simulink model "ndtm_V2"  (R2018b)
settings: configuration reference "Physics" (kept outside this file)
model workspace (MAT data in the model file):
  x0_initialstates = [0 0 0 0 0 0]
undefined symbols (not defined in the file): F0z, h, INIT__initialvalues__Vehicle_InitialPitchRate_radps, INIT__initialvalues__Vehicle_InitialRollRate_radps, INIT__initialvalues__Vehicle_InitialVelocity_mps__1, INIT__initialvalues__Vehicle_InitialVelocity_mps__2, INIT__initialvalues__Vehicle_InitialVelocity_mps__3, INIT__initialvalues__Vehicle_InitialYawRate_radps, SUS__Antisway__c_AntiSwayTSpringFrRe_Nmprad__1, SUS__Antisway__c_AntiSwayTSpringFrRe_Nmprad__2, SUS__Antisway__phi_AntiSwayNeutralAngleFrRe_rad__1, SUS__Antisway__phi_AntiSwayNeutralAngleFrRe_rad__2, SUS__Antisway__r_AntiSwayArmRadiusFrRe_m__1, SUS__Antisway__r_AntiSwayArmRadiusFrRe_m__2, SUS__Compliance__Cz_DamperRateFrRe_Nspm__1, SUS__Compliance__Cz_DamperRateFrRe_Nspm__2, SUS__Compliance__cz_SpringRateFrRe_Npm__1, SUS__Compliance__cz_SpringRateFrRe_Npm__2, SUS__Compliance__F0z_SpringPreloadFrRe_N__1, SUS__Compliance__F0z_SpringPreloadFrRe_N__2, SUS__Compliance__h_InertialFrameOffset_COGtoAxle_m, SUS__Kinematics__k_CamberATSteerCenterF__1, SUS__Kinematics__k_CamberATSteerCenterF__2, SUS__Kinematics__k_CamberVSHeightFrRe__1, SUS__Kinematics__k_CamberVSHeightFrRe__2, SUS__Kinematics__k_CasterATSteerCenterF__1, SUS__Kinematics__k_CasterATSteerCenterF__2, SUS__Kinematics__k_CasterVSHeightFrRe__1, SUS__Kinematics__k_CasterVSHeightFrRe__2, SUS__Kinematics__k_RollSteerVSHeightFrRe_radpm__1, SUS__Kinematics__k_RollSteerVSHeightFrRe_radpm__2, SUS__Kinematics__nu0_ToeATSteerCenterFrRe_rad__1, SUS__Kinematics__nu0_ToeATSteerCenterFrRe_rad__2, tireFL__SCALING__LFZO, tireFR__SCALING__LFZO, tireRL__SCALING__LFZO, tireRR__SCALING__LFZO, VEH, VEH__Aerodynamics__beta_wind_end_rad, VEH__Aerodynamics__beta_wind_start_rad, VEH__Aerodynamics__beta_wind_step_rad, VEH__Aerodynamics__cl_LongitudinalLift, VEH__Aerodynamics__Cs_LatDragCoeff_end, VEH__Aerodynamics__Cs_LatDragCoeff_start, VEH__Aerodynamics__Cs_LatDragCoeff_step, VEH__Aerodynamics__Cym_DragYawMomentCoeff_end, VEH__Aerodynamics__Cym_DragYawMomentCoeff_start, VEH__Aerodynamics__Cym_DragYawMomentCoeff_step, VEH__Environment__a_Gravity_mps2, VEH__Tires__p_Tires_pa__1, VEH__Tires__p_Tires_pa__2, VEH__Tires__p_Tires_pa__3, VEH__Tires__p_Tires_pa__4, VEH__VehicleData__l_WheelbaseF_m, VEH__VehicleData__l_WheelbaseTotal_m, VEH__VehicleData__m_Vehicle_kg, VEH__VehicleData__w_GeomCenterlineToCOG_m, VEH__VehicleData__w_TrackF_m, VEH__VehicleData__w_TrackR_m
libraries: vehdynlibsuspension x7, vehdynlibtire x4, vehdynlibtire_TUM x4, autolibutils x2, sharedtransform x2, vehdynlibeom_TUM x1
(part 1 of 4)
settings Model: DataDictionary=vehicleparameters_vehdynsim.sldd  ModifiedByFormat=The MathWorks, Inc.  ParameterArgumentNames=x0_initialstates  OrderedModelArguments=off  Creator=The MathWorks, Inc.  LastModifiedBy=The MathWorks, Inc.

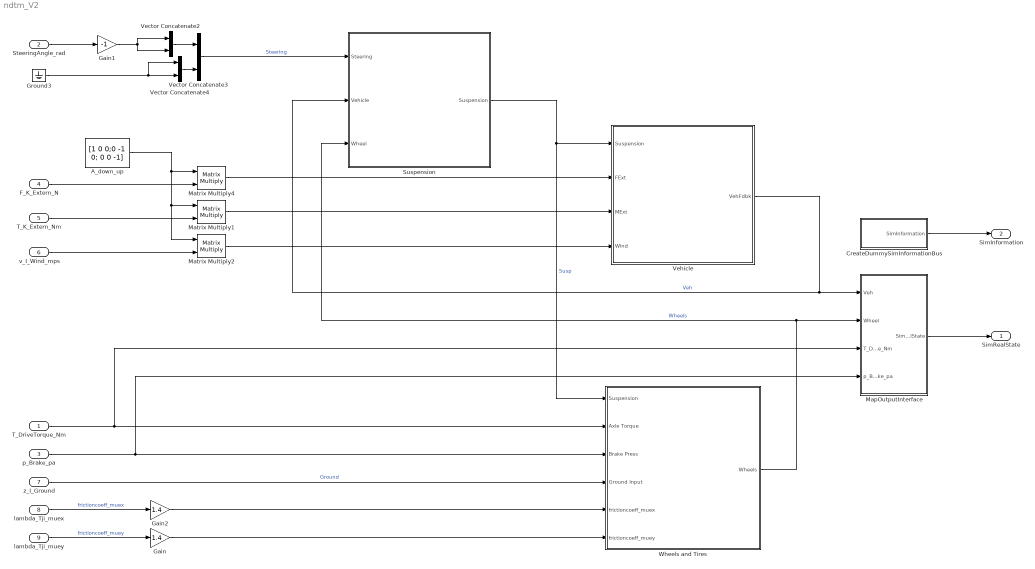
== system ndtm_V2 ==
  T_DriveTorque_Nm : Inport
  SteeringAngle_rad : Inport  Port=2
  p_Brake_pa : Inport  Port=3
  F_K_Extern_N : Inport  Port=4  PortDimensions=3
  T_K_Extern_Nm : Inport  Port=5  PortDimensions=3
  v_I_Wind_mps : Inport  Port=6  PortDimensions=3
  z_I_Ground : Inport  Port=7  PortDimensions=4
  lambda_Tji_muex : Inport  Port=8  PortDimensions=4
  lambda_Tji_muey : Inport  Port=9  PortDimensions=4
  A_down_up : Constant  Value=[1 0 0;0 -1 0; 0 0 -1]
  CreateDummySimInformationBus : Subsystem
  Gain : Gain  Gain=1.4
  Gain1 : Gain  Gain=-1
  Gain2 : Gain  Gain=1.4
  Ground3 : Ground
  MapOutputInterface : Subsystem
  Matrix Multiply1 : Product  Multiplication=Matrix(*)
  Matrix Multiply2 : Product  Multiplication=Matrix(*)
  Matrix Multiply4 : Product  Multiplication=Matrix(*)
  Suspension : Subsystem  VariantControlMode=Label  Variant=on  LabelModeActiveChoice=1
      mask Display:
      | switch str2num(get_param(gcb,'ActiveVariant'))
      |     case 1
      |         image('suspdw.png');
      |     case 2
      |         image([imread('suspindmap.png');imread('suspsamap.png')]);
      |     case 3
      |          image([imread('suspmacp.png');imread('suspsacoil.png')]);
      |     case 4
      |          image('suspmacp.png');
      |     case 5
      |          image('suspindmap.png');
      | end
  Vector Concatenate2 : Concatenate
  Vector Concatenate3 : Concatenate
  Vector Concatenate4 : Concatenate
  Vehicle : Subsystem
      mask Display: image('6dofcar.png');
  Wheels and Tires : Subsystem
      mask Display: image('wheel3dof.png')
  SimRealState : Outport  OutDataTypeStr=Bus: SimRealState
  SimInformation : Outport  Port=2  OutDataTypeStr=Bus: SimInformation
  wires:
  Vehicle/1(VehFdbk) -> Suspension/2(Vehicle), MapOutputInterface/1(Veh)  "Veh"
  Vector Concatenate3/1 -> Suspension/1(Steering)  "Steering"
  Suspension/1(Suspension) -> Vehicle/1(Suspension), Wheels and Tires/1(Suspension)  "Susp"
  Wheels and Tires/1(Wheels) -> MapOutputInterface/2(Wheel), Suspension/3(Wheel)  "Wheels"
  z_I_Ground/1 -> Wheels and Tires/4(Ground Input)  "Ground"
  p_Brake_pa/1 -> Wheels and Tires/3(Brake Press), MapOutputInterface/4("p_Brake_pa ")
  Ground3/1 -> Vector Concatenate4/1, Vector Concatenate4/2
  lambda_Tji_muey/1 -> Gain/1  "frictioncoeff_muey"
  Gain1/1 -> Vector Concatenate2/2, Vector Concatenate2/1
  Matrix Multiply4/1 -> Vehicle/2(FExt)
  Vector Concatenate2/1 -> Vector Concatenate3/1
  Matrix Multiply2/1 -> Vehicle/4(Wind)
  Matrix Multiply1/1 -> Vehicle/3(MExt)
  Vector Concatenate4/1 -> Vector Concatenate3/2
  T_DriveTorque_Nm/1 -> Wheels and Tires/2(Axle Torque), MapOutputInterface/3(T_DriveTorque_Nm)
  CreateDummySimInformationBus/1(SimInformation) -> SimInformation/1
  MapOutputInterface/1(SimRealState) -> SimRealState/1
  SteeringAngle_rad/1 -> Gain1/1
  lambda_Tji_muex/1 -> Gain2/1  "frictioncoeff_muex"
  F_K_Extern_N/1 -> Matrix Multiply4/2
  A_down_up/1 -> Matrix Multiply2/1, Matrix Multiply1/1, Matrix Multiply4/1
  T_K_Extern_Nm/1 -> Matrix Multiply1/2
  v_I_Wind_mps/1 -> Matrix Multiply2/2
  Gain2/1 -> Wheels and Tires/5(frictioncoeff_muex)
  Gain/1 -> Wheels and Tires/6(frictioncoeff_muey)

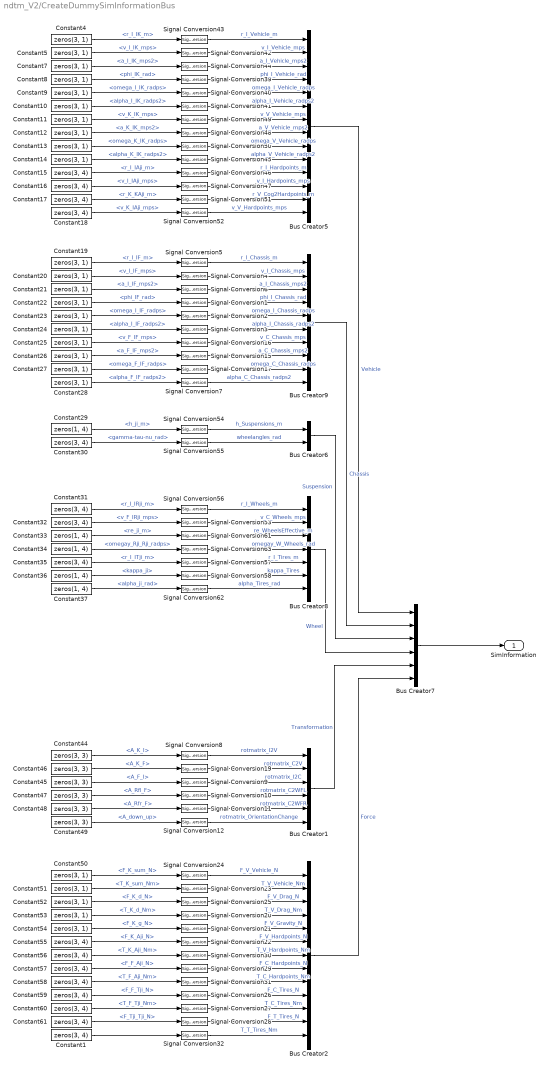
== system ndtm_V2/CreateDummySimInformationBus ==
  Bus Creator1 : BusCreator  Inputs=6  OutDataTypeStr=Bus: Transformation
      settings: InheritFromInputs=off
  Bus Creator2 : BusCreator  Inputs=13  OutDataTypeStr=Bus: Force
      settings: InheritFromInputs=off
  Bus Creator5 : BusCreator  Inputs=14  OutDataTypeStr=Bus: Vehicle
      settings: InheritFromInputs=off
  Bus Creator6 : BusCreator  Inputs=2  OutDataTypeStr=Bus: Suspension
      settings: InheritFromInputs=off
  Bus Creator7 : BusCreator  Inputs=6  OutDataTypeStr=Bus: SimInformation
      settings: InheritFromInputs=off
  Bus Creator8 : BusCreator  Inputs=7  OutDataTypeStr=Bus: Wheel
      settings: InheritFromInputs=off
  Bus Creator9 : BusCreator  Inputs=10  OutDataTypeStr=Bus: Chassis
      settings: InheritFromInputs=off
  Constant{1,15..18,30..32,35,55..61} (16 alike) : Constant  Value=zeros(3, 4)
  Constant{4..5,7..14,19..28,50..54} (25 alike) : Constant  Value=zeros(3, 1)
  Constant{29,33..34,36..37} (5 alike) : Constant  Value=zeros(1, 4)
  Constant{44..49} (6 alike) : Constant  Value=zeros(3, 3)
  Signal Conversion{1..12,15..17,19..32,39..58,61..63} (52 alike) : SignalConversion  OverrideOpt=off
  SimInformation : Outport  OutDataTypeStr=Bus: SimInformation
  wires:
  Signal Conversion46/1 -> Bus Creator5/11  "r_I_Hardpoints_m"
  Signal Conversion26/1 -> Bus Creator2/10  "F_C_Tires_N"
  Signal Conversion45/1 -> Bus Creator5/10  "alpha_V_Vehicle_radps2"
  Constant33/1 -> Signal Conversion61/1  "<re_ji_m>"
  Signal Conversion15/1 -> Bus Creator9/8  "a_C_Chassis_mps2"
  Signal Conversion58/1 -> Bus Creator8/6  "kappa_Tires"
  Constant60/1 -> Signal Conversion27/1  "<T_F_Tji_Nm>"
  Signal Conversion5/1 -> Bus Creator9/1  "r_I_Chassis_m"
  Signal Conversion17/1 -> Bus Creator9/9  "omega_C_Chassis_radps"
  Signal Conversion8/1 -> Bus Creator1/1  "rotmatrix_I2V"
  Constant13/1 -> Signal Conversion50/1  "<omega_K_IK_radps>"
  Constant24/1 -> Signal Conversion3/1  "<alpha_I_IF_radps2>"
  Signal Conversion16/1 -> Bus Creator9/7  "v_C_Chassis_mps"
  Signal Conversion23/1 -> Bus Creator2/2  "T_V_Vehicle_Nm"
  Signal Conversion3/1 -> Bus Creator9/6  "alpha_I_Chassis_radps2"
  Bus Creator5/1 -> Bus Creator7/1  "Vehicle"
  Signal Conversion32/1 -> Bus Creator2/13  "T_T_Tires_Nm"
  Signal Conversion39/1 -> Bus Creator5/4  "phi_I_Vehicle_rad"
  Signal Conversion29/1 -> Bus Creator2/8  "F_C_Hardpoints_N"
  Constant25/1 -> Signal Conversion16/1  "<v_F_IF_mps>"
  Signal Conversion43/1 -> Bus Creator5/1  "r_I_Vehicle_m"
  Constant47/1 -> Signal Conversion10/1  "<A_Rfl_F>"
  Constant9/1 -> Signal Conversion40/1  "<omega_I_IK_radps>"
  Constant26/1 -> Signal Conversion15/1  "<a_F_IF_mps2>"
  Constant27/1 -> Signal Conversion17/1  "<omega_F_IF_radps>"
  Signal Conversion10/1 -> Bus Creator1/4  "rotmatrix_C2WFL"
  Signal Conversion19/1 -> Bus Creator1/2  "rotmatrix_C2V"
  Constant7/1 -> Signal Conversion44/1  "<a_I_IK_mps2>"
  Bus Creator8/1 -> Bus Creator7/4  "Wheel"
  Signal Conversion9/1 -> Bus Creator1/3  "rotmatrix_I2C"
  Signal Conversion31/1 -> Bus Creator2/9  "T_C_Hardpoints_Nm"
  Signal Conversion62/1 -> Bus Creator8/7  "alpha_Tires_rad"
  Signal Conversion30/1 -> Bus Creator2/7  "T_V_Hardpoints_Nm"
  Signal Conversion48/1 -> Bus Creator5/8  "a_V_Vehicle_mps2"
  Signal Conversion54/1 -> Bus Creator6/1  "h_Suspensions_m"
  Signal Conversion56/1 -> Bus Creator8/1  "r_I_Wheels_m"
  Signal Conversion7/1 -> Bus Creator9/10  "alpha_C_Chassis_radps2"
  Signal Conversion12/1 -> Bus Creator1/6  "rotmatrix_OrientationChange"
  Signal Conversion21/1 -> Bus Creator2/5  "F_V_Gravity_N"
  Signal Conversion53/1 -> Bus Creator8/2  "v_C_Wheels_mps"
  Signal Conversion22/1 -> Bus Creator2/6  "F_V_Hardpoints_N"
  Signal Conversion27/1 -> Bus Creator2/11  "T_C_Tires_Nm"
  Signal Conversion51/1 -> Bus Creator5/13  "r_V_Cog2Hardpoints_m"
  Constant28/1 -> Signal Conversion7/1  "<alpha_F_IF_radps2>"
  Signal Conversion55/1 -> Bus Creator6/2  "wheelangles_rad"
  Signal Conversion57/1 -> Bus Creator8/5  "r_I_Tires_m"
  Signal Conversion4/1 -> Bus Creator9/2  "v_I_Chassis_mps"
  Bus Creator2/1 -> Bus Creator7/6  "Force"
  Signal Conversion20/1 -> Bus Creator2/4  "T_V_Drag_Nm"
  Signal Conversion40/1 -> Bus Creator5/5  "omega_I_Vehicle_radps"
  Bus Creator1/1 -> Bus Creator7/5  "Transformation"
  Signal Conversion41/1 -> Bus Creator5/6  "alpha_I_Vehicle_radps2"
  Bus Creator9/1 -> Bus Creator7/2  "Chassis"
  Signal Conversion6/1 -> Bus Creator9/3  "a_I_Chassis_mps2"
  Bus Creator6/1 -> Bus Creator7/3  "Suspension"
  Signal Conversion61/1 -> Bus Creator8/3  "re_WheelsEffective_m"
  Signal Conversion44/1 -> Bus Creator5/3  "a_I_Vehicle_mps2"
  Signal Conversion42/1 -> Bus Creator5/2  "v_I_Vehicle_mps"
  Signal Conversion63/1 -> Bus Creator8/4  "omegay_W_Wheels_rad"
  Constant31/1 -> Signal Conversion56/1  "<r_I_IRji_m>"
  Signal Conversion49/1 -> Bus Creator5/7  "v_V_Vehicle_mps"
  Signal Conversion28/1 -> Bus Creator2/12  "F_T_Tires_N"
  Signal Conversion11/1 -> Bus Creator1/5  "rotmatrix_C2WFR"
  Signal Conversion50/1 -> Bus Creator5/9  "omega_V_Vehicle_radps"
  Signal Conversion24/1 -> Bus Creator2/1  "F_V_Vehicle_N"
  Constant19/1 -> Signal Conversion5/1  "<r_I_IF_m>"
  Constant22/1 -> Signal Conversion1/1  "<phi_IF_rad>"
  Constant11/1 -> Signal Conversion49/1  "<v_K_IK_mps>"
  Constant58/1 -> Signal Conversion31/1  "<T_F_Aji_Nm>"
  Constant20/1 -> Signal Conversion4/1  "<v_I_IF_mps>"
  Constant44/1 -> Signal Conversion8/1  "<A_K_I>"
  Constant36/1 -> Signal Conversion58/1  "<kappa_ji>"
  Constant32/1 -> Signal Conversion53/1  "<v_F_IRji_mps>"
  Constant8/1 -> Signal Conversion39/1  "<phi_IK_rad>"
  Signal Conversion2/1 -> Bus Creator9/5  "omega_I_Chassis_radps"
  Constant5/1 -> Signal Conversion42/1  "<v_I_IK_mps>"
  Constant10/1 -> Signal Conversion41/1  "<alpha_I_IK_radps2>"
  Constant4/1 -> Signal Conversion43/1  "<r_I_IK_m>"
  Constant29/1 -> Signal Conversion54/1  "<h_ji_m>"
  Constant1/1 -> Signal Conversion32/1
  Constant35/1 -> Signal Conversion57/1  "<r_I_ITji_m>"
  Signal Conversion47/1 -> Bus Creator5/12  "v_I_Hardpoints_mps"
  Constant57/1 -> Signal Conversion29/1  "<F_F_Aji_N>"
  Constant48/1 -> Signal Conversion11/1  "<A_Rfr_F>"
  Constant50/1 -> Signal Conversion24/1  "<F_K_sum_N>"
  Constant53/1 -> Signal Conversion20/1  "<T_K_d_Nm>"
  Constant49/1 -> Signal Conversion12/1  "<A_down_up>"
  Constant51/1 -> Signal Conversion23/1  "<T_K_sum_Nm>"
  Constant12/1 -> Signal Conversion48/1  "<a_K_IK_mps2>"
  Constant15/1 -> Signal Conversion46/1  "<r_I_IAji_m>"
  Constant54/1 -> Signal Conversion21/1  "<F_K_g_N>"
  Constant17/1 -> Signal Conversion51/1  "<r_K_KAji_m>"
  Constant55/1 -> Signal Conversion22/1  "<F_K_Aji_N>"
  Constant21/1 -> Signal Conversion6/1  "<a_I_IF_mps2>"
  Constant52/1 -> Signal Conversion25/1  "<F_K_d_N>"
  Constant30/1 -> Signal Conversion55/1  "<gamma-tau-nu_rad>"
  Constant14/1 -> Signal Conversion45/1  "<alpha_K_IK_radps2>"
  Constant18/1 -> Signal Conversion52/1  "<v_K_IAji_mps>"
  Constant59/1 -> Signal Conversion26/1  "<F_F_Tji_N>"
  Constant61/1 -> Signal Conversion28/1  "<F_Tji_Tji_N>"
  Constant56/1 -> Signal Conversion30/1  "<T_K_Aji_Nm>"
  Constant37/1 -> Signal Conversion62/1  "<alpha_ji_rad>"
  Constant34/1 -> Signal Conversion63/1  "<omegay_Rji_Rji_radps>"
  Constant45/1 -> Signal Conversion9/1  "<A_F_I>"
  Signal Conversion1/1 -> Bus Creator9/4  "phi_I_Chassis_rad"
  Signal Conversion52/1 -> Bus Creator5/14  "v_V_Hardpoints_mps"
  Constant46/1 -> Signal Conversion19/1  "<A_K_F>"
  Constant23/1 -> Signal Conversion2/1  "<omega_I_IF_radps>"
  Constant16/1 -> Signal Conversion47/1  "<v_I_IAji_mps>"
  Signal Conversion25/1 -> Bus Creator2/3  "F_V_Drag_N"
  Bus Creator7/1 -> SimInformation/1

== system ndtm_V2/MapOutputInterface ==
  Veh : Inport
  Wheel : Inport  Port=2
  T_DriveTorque_Nm : Inport  Port=3
  "p_Brake_pa " : Inport  Port=4
  Bus Creator3 : BusCreator  Inputs=32  OutDataTypeStr=Bus: SimRealState
  Demux{,1..4} (5 alike) : Demux  Outputs=3
  Demux{5..8} (4 alike) : Demux
  Ground : Ground
  Vehicle Routing : Subsystem
  Wheel Routing : Subsystem
  SimRealState : Outport  OutDataTypeStr=Bus: SimRealState
  wires:
  Ground/1 -> Demux5/1
  Demux3/2 -> Bus Creator3/11  "dTheta_radps"
  Demux1/1 -> Bus Creator3/4  "phi_rad"
  Demux3/1 -> Bus Creator3/10  "dPhi_radps"
  Demux1/2 -> Bus Creator3/5  "theta_rad"
  Demux5/4 -> Bus Creator3/23  "dnWheelRR_radps2"
  Demux6/1 -> Bus Creator3/16  "nWheelFL_radps"
  Demux4/3 -> Bus Creator3/15  "az_mps2"
  Vehicle Routing/3(Cgxyzdot) -> Demux2/1
  Demux/3 -> Bus Creator3/3  "z_m"
  Demux2/3 -> Bus Creator3/9  "vz_mps"
  Bus Creator3/1 -> SimRealState/1
  Vehicle Routing/2(angles) -> Demux1/1
  Vehicle Routing/5(Cgaxyz) -> Demux4/1
  Demux5/2 -> Bus Creator3/21  "dnWheelFR_radps2"
  Wheel Routing/2(SteeringWheelAngle) -> Bus Creator3/24  "DeltaWheel_rad"
  Demux5/1 -> Bus Creator3/20  "dnWheelFL_radps2"
  Wheel/1 -> Wheel Routing/1(Wheel)
  Demux6/4 -> Bus Creator3/19  "nWheelRR_radps"
  Demux5/3 -> Bus Creator3/22  "dnWheelRL_radps2"
  Veh/1 -> Vehicle Routing/1(Veh)
  Demux3/3 -> Bus Creator3/12  "dPsi_radps"
  Vehicle Routing/4(pqr) -> Demux3/1
  Demux4/2 -> Bus Creator3/14  "ay_mps2"
  Demux6/2 -> Bus Creator3/17  "nWheelFR_radps"
  Demux6/3 -> Bus Creator3/18  "nWheelRL_radps"
  Wheel Routing/1(omega) -> Demux6/1
  Vehicle Routing/1(CgXYZ) -> Demux/1
  Demux/2 -> Bus Creator3/2  "y_m"
  Demux/1 -> Bus Creator3/1  "x_m"
  Demux1/3 -> Bus Creator3/6  "psi_rad"
  Demux2/2 -> Bus Creator3/8  "vy_mps"
  Demux2/1 -> Bus Creator3/7  "vx_mps"
  Demux4/1 -> Bus Creator3/13  "ax_mps2"
  T_DriveTorque_Nm/1 -> Demux7/1
  Demux7/4 -> Bus Creator3/28  "T_DriveTorqueRR_Nm"
  Demux8/2 -> Bus Creator3/30  "p_BrakePressureFR_pa"
  Demux8/4 -> Bus Creator3/32  "p_BrakePressureRR_pa"
  "p_Brake_pa "/1 -> Demux8/1
  Demux8/1 -> Bus Creator3/29  "p_BrakePressureFL_pa"
  Demux7/3 -> Bus Creator3/27  "T_DriveTorqueRL_Nm"
  Demux8/3 -> Bus Creator3/31  "p_BrakePressureRL_pa"
  Demux7/1 -> Bus Creator3/25  "T_DriveTorqueFL_Nm"
  Demux7/2 -> Bus Creator3/26  "T_DriveTorqueFR_Nm"

== system ndtm_V2/Suspension ==
  Steering : Inport
  Vehicle : Inport  Port=2
  Wheel : Inport  Port=3
  Double Wishbone Suspension : Subsystem  VariantControl=1
      mask Display: image('suspdw.png');
  Independent Mapped Front Suspension Mapped Solid Axle Rear Suspension : Subsystem  VariantControl=2
      mask Display: image([imread('suspindmap.png');imread('suspsamap.png')]);
  MacPherson Front Suspension Solid Axle Rear Suspension : Subsystem  VariantControl=3
      mask Display: image([imread('suspmacp.png');imread('suspsacoil.png')]);
  MacPherson Suspension : Subsystem  VariantControl=4
      mask Display: image('suspmacp.png');
  Mapped Suspension : Subsystem  VariantControl=5
      mask Display: image('suspindmap.png');
  Suspension : Outport

== system ndtm_V2/Vehicle ==
  Suspension : Inport
  FExt : Inport  Port=2
  MExt : Inport  Port=3
  Wind : Inport  Port=4
  Bus Selector3 : BusSelector  OutputSignals=Veh.F,Veh.M
  Terminator{,1..5} (6 alike) : Terminator
  Vehicle Body 6DOF - TUM : vehdynlibeom_TUM/Vehicle Body 6DOF  m=VEH__VehicleData__m_Vehicle_kg  a=VEH__VehicleData__l_WheelbaseF_m  b=VEH__VehicleData__l_WheelbaseTotal_m - VEH__VehicleData__l_WheelbaseF_m  d=- VEH__VehicleData__w_GeomCenterlineToCOG_m  h=VEH__VehicleData__h_AxlePlaneToCOG_m  Xe_o=x0_initialstates(1:3)  xbdot_o=[INIT__initialvalues__Vehicle_InitialVelocity_mps__1, - INIT__initialvalues__Vehicle_InitialVelocity_mps__2, - INIT__initialvalues__Vehicle_InitialVelocity_mps__3]  eul_o=x0_initialstates(4:6)  p_o=[INIT__initialvalues__Vehicle_InitialRollRate_radps, - INIT__initialvalues__Vehicle_InitialPitchRate_radps, - INIT__initialvalues__Vehicle_InitialYawRate_radps]  Iveh=[VEH__VehicleData__I_K_Vehicle_kgm2__11, VEH__VehicleData__I_K_Vehicle_kgm2__12, VEH__VehicleData__I_K_Vehicle_kgm2__13; VEH__VehicleData__I_K_Vehicle_kgm2__21, VEH__VehicleData__I_K_Vehicle_kgm2__22, VEH__VehicleData__I_K_Vehicle_kgm2__23; VEH__VehicleData__I_K_Vehicle_kgm2__31, VEH__VehicleData__I_K_Vehicle_kgm2__32, VEH__VehicleData__I_K_Vehicle_kgm2__33]  w=[VEH__VehicleData__w_TrackF_m, VEH__VehicleData__w_TrackR_m]  z1m=0  z1R=[-.25,.125,.15]  z1I=[1.4,-.2,.1;-.2,1.4,.1;.1,.1,2.25].*0  z2m=0  z2R=[1.4,0,.8]  z2I=[1.4,-.2,.1;-.2,1.4,.1;.1,.1,2.25].*0  z3m=0  z3R=[.75,-.5,.4]  z3I=[5,-.1,-2;-2,9,.1;-.1,.1,6].*0  z4m=0  z4R=[.75,.5,.4]  z4I=[5,-.1,-2;-2,9,.1;-.1,.1,6].*0  z5m=0  z5R=[1.25,-.5,.4]  z5I=[5,-.1,-2;-2,9,.1;-.1,.1,6].*0  z6m=0  z6R=[1.25,-.5,.4]  z6I=[5,-.1,-2;-2,9,.1;-.1,.1,6].*0  z7m=0  z7R=[2,0,.25]  z7I=[1.4,-.2,.1;-.2,1.4,.1;.1,.1,2.25].*0  Af=VEH__Aerodynamics__A_LongitudinalDrag_m2  Cd=VEH__Aerodynamics__cw_LongitudinalDrag  Cl=abs(VEH__Aerodynamics__cl_LongitudinalLift)  Cpm=VEH__Aerodynamics__cpm_LongDragPitchMomentCoeff  beta_w=[VEH__Aerodynamics__beta_wind_start_rad:VEH__Aerodynamics__beta_wind_step_rad:VEH__Aerodynamics__beta_wind_end_rad]  Cs=[VEH__Aerodynamics__Cs_LatDragCoeff_start:VEH__Aerodynamics__Cs_LatDragCoeff_step:VEH__Aerodynamics__Cs_LatDragCoeff_end]  Cym=[VEH__Aerodynamics__Cym_DragYawMomentCoeff_start:VEH__Aerodynamics__Cym_DragYawMomentCoeff_step:VEH__Aerodynamics__Cym_DragYawMomentCoeff_end]  sign_cl=sign(VEH__Aerodynamics__cl_LongitudinalLift)  Pabs=VEH__Environment__p_Air_Pa  Tair=VEH__Environment__T_Air_K  g=VEH__Environment__a_Gravity_mps2  xdot_tol=VEH__Simulation__Sim_LongVelTolerance_mps  longOff=VEH__Simulation__Sim_LongOff_m  latOff=VEH__Simulation__Sim_LatOff_m  vertOff=VEH__Simulation__Sim_VertOff_m  aMode=2
  VehFdbk : Outport
  wires:
  Vehicle Body 6DOF - TUM/4 -> Terminator2/1
  MExt/1 -> Vehicle Body 6DOF - TUM/4
  Vehicle Body 6DOF - TUM/7 -> Terminator5/1
  Vehicle Body 6DOF - TUM/5 -> Terminator3/1
  Vehicle Body 6DOF - TUM/2 -> Terminator/1
  Suspension/1 -> Bus Selector3/1
  FExt/1 -> Vehicle Body 6DOF - TUM/3
  Vehicle Body 6DOF - TUM/6 -> Terminator4/1
  Bus Selector3/1 -> Vehicle Body 6DOF - TUM/1  "<F>"
  Vehicle Body 6DOF - TUM/1 -> VehFdbk/1  "VehFdbk"
  Bus Selector3/2 -> Vehicle Body 6DOF - TUM/2  "<M>"
  Wind/1 -> Vehicle Body 6DOF - TUM/5
  Vehicle Body 6DOF - TUM/3 -> Terminator1/1

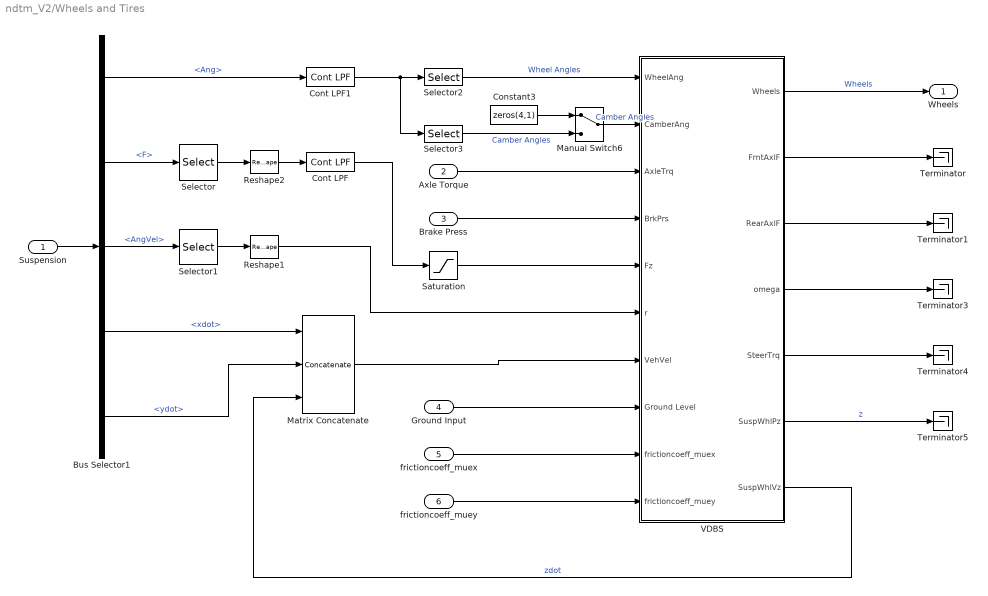
== system ndtm_V2/Wheels and Tires ==
  Suspension : Inport
  Axle Torque : Inport  Port=2
  Brake Press : Inport  Port=3  Unit=Pa
  Ground Input : Inport  Port=4
  frictioncoeff_muex : Inport  Port=5  PortDimensions=4
  frictioncoeff_muey : Inport  Port=6  PortDimensions=4
  Bus Selector1 : BusSelector  OutputSignals=Whl.Ang,Whl.F,Whl.AngVel,Whl.xdot,Whl.ydot
  Constant3 : Constant  Value=zeros(4,1)
  Cont LPF : autolibutils/Cont LPF  wc=100*2*pi  aMode=2
      settings: SourceProductName=Powertrain Blockset  SourceProductBaseCode=PW
  Cont LPF1 : autolibutils/Cont LPF  wc=100*2*pi  aMode=2
      settings: SourceProductName=Powertrain Blockset  SourceProductBaseCode=PW
  Manual Switch6 : ManualSwitch
  Matrix Concatenate : Concatenate  NumInputs=3  Mode=Multidimensional array
  Reshape1 : Reshape
  Reshape2 : Reshape
  Saturation : Saturate  UpperLimit=inf  LowerLimit=-10*9.81*2000  ZeroCross=off
  Selector : Selector  NumberOfDimensions=2  InputPortWidth=3  IndexOptions=Index vector (dialog),Select all  Indices=[3],1  OutputSizes=1,1
  Selector1 : Selector  NumberOfDimensions=2  InputPortWidth=1  IndexOptions=Index vector (dialog),Select all  Indices=[3],1  OutputSizes=1,1
  Selector2 : Selector  NumberOfDimensions=2  InputPortWidth=3  IndexOptions=Index vector (dialog),Select all  Indices=3,1  OutputSizes=1,1
  Selector3 : Selector  NumberOfDimensions=2  InputPortWidth=3  IndexOptions=Index vector (dialog),Select all  Indices=1,1  OutputSizes=1,1
  Terminator{,1,3..5} (5 alike) : Terminator
  VDBS : Subsystem  VariantControl=0
  Wheels : Outport
  wires:
  VDBS/1(Wheels) -> Wheels/1  "Wheels"
  Bus Selector1/2 -> Selector/1  "<F>"
  VDBS/2(FrntAxlF) -> Terminator/1
  VDBS/3(RearAxlF) -> Terminator1/1
  VDBS/4(omega) -> Terminator3/1
  VDBS/5(SteerTrq) -> Terminator4/1
  Selector1/1 -> Reshape1/1
  Matrix Concatenate/1 -> VDBS/7(VehVel)
  Axle Torque/1 -> VDBS/3(AxleTrq)
  Selector2/1 -> VDBS/1(WheelAng)  "Wheel Angles"
  Constant3/1 -> Manual Switch6/1
  Manual Switch6/1 -> VDBS/2(CamberAng)  "Camber Angles"
  Selector/1 -> Reshape2/1
  Saturation/1 -> VDBS/5(Fz)
  Ground Input/1 -> VDBS/8(Ground Level)
  VDBS/7(SuspWhlVz) -> Matrix Concatenate/3  "zdot"
  Bus Selector1/1 -> Cont LPF1/1  "<Ang>"
  Selector3/1 -> Manual Switch6/2  "Camber Angles"
  Suspension/1 -> Bus Selector1/1
  Bus Selector1/4 -> Matrix Concatenate/1  "<xdot>"
  Bus Selector1/5 -> Matrix Concatenate/2  "<ydot>"
  VDBS/6(SuspWhlPz) -> Terminator5/1  "z"
  Reshape2/1 -> Cont LPF/1
  Bus Selector1/3 -> Selector1/1  "<AngVel>"
  Reshape1/1 -> VDBS/6(r)
  Brake Press/1 -> VDBS/4(BrkPrs)
  frictioncoeff_muex/1 -> VDBS/9(frictioncoeff_muex)
  Cont LPF/1 -> Saturation/1
  Cont LPF1/1 -> Selector3/1, Selector2/1
  frictioncoeff_muey/1 -> VDBS/10(frictioncoeff_muey)

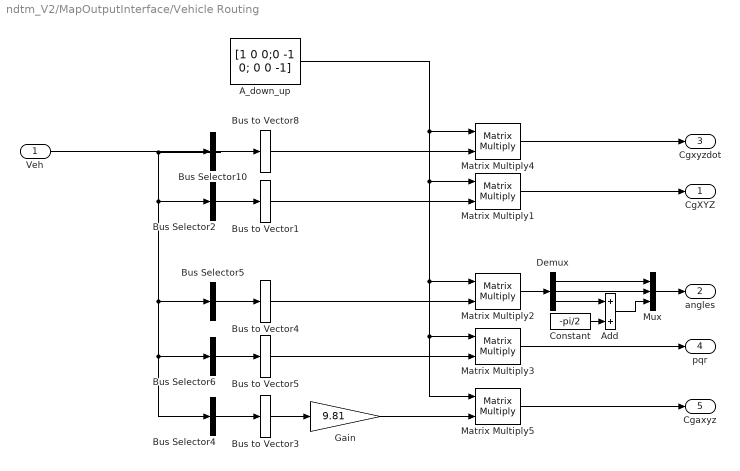
== system ndtm_V2/MapOutputInterface/Vehicle Routing ==
  Veh : Inport
  A_down_up : Constant  Value=[1 0 0;0 -1 0; 0 0 -1]
  Add : Sum
  Bus Selector10 : BusSelector  OutputSignals=BdyFrm.Cg.Vel.xdot,BdyFrm.Cg.Vel.ydot,BdyFrm.Cg.Vel.zdot  OutputAsBus=on
  Bus Selector2 : BusSelector  OutputSignals=InertFrm.Cg.Disp.X,InertFrm.Cg.Disp.Y,InertFrm.Cg.Disp.Z  OutputAsBus=on
  Bus Selector4 : BusSelector  OutputSignals=BdyFrm.Cg.Acc.ax,BdyFrm.Cg.Acc.ay,BdyFrm.Cg.Acc.az  OutputAsBus=on
  Bus Selector5 : BusSelector  OutputSignals=InertFrm.Cg.Ang.phi,InertFrm.Cg.Ang.theta,InertFrm.Cg.Ang.psi  OutputAsBus=on
  Bus Selector6 : BusSelector  OutputSignals=BdyFrm.Cg.AngVel.p,BdyFrm.Cg.AngVel.q,BdyFrm.Cg.AngVel.r  OutputAsBus=on
  Bus to Vector{1,3..5,8} (5 alike) : BusToVector
  Constant : Constant  Value=-pi/2
  Demux : Demux  Outputs=3
  Gain : Gain  Gain=9.81
  Matrix Multiply{1..5} (5 alike) : Product  Multiplication=Matrix(*)
  Mux : Mux  Inputs=3
  CgXYZ : Outport
  angles : Outport  Port=2
  Cgxyzdot : Outport  Port=3
  pqr : Outport  Port=4
  Cgaxyz : Outport  Port=5
  wires:
  Bus Selector5/1 -> Bus to Vector4/1
  Bus Selector6/1 -> Bus to Vector5/1
  Bus Selector2/1 -> Bus to Vector1/1
  Bus Selector4/1 -> Bus to Vector3/1
  Bus Selector10/1 -> Bus to Vector8/1
  Veh/1 -> Bus Selector2/1, Bus Selector5/1, Bus Selector6/1, Bus Selector4/1, Bus Selector10/1
  A_down_up/1 -> Matrix Multiply4/1, Matrix Multiply5/1, Matrix Multiply3/1, Matrix Multiply2/1, Matrix Multiply1/1
  Matrix Multiply4/1 -> Cgxyzdot/1
  Matrix Multiply3/1 -> pqr/1
  Matrix Multiply5/1 -> Cgaxyz/1
  Bus to Vector8/1 -> Matrix Multiply4/2
  Bus to Vector1/1 -> Matrix Multiply1/2
  Bus to Vector4/1 -> Matrix Multiply2/2
  Bus to Vector5/1 -> Matrix Multiply3/2
  Add/1 -> Mux/3
  Demux/3 -> Add/1
  Demux/2 -> Mux/2
  Mux/1 -> angles/1
  Demux/1 -> Mux/1
  Constant/1 -> Add/2
  Matrix Multiply2/1 -> Demux/1
  Matrix Multiply1/1 -> CgXYZ/1
  Bus to Vector3/1 -> Gain/1
  Gain/1 -> Matrix Multiply5/2

== system ndtm_V2/MapOutputInterface/Wheel Routing ==
  Wheel : Inport
  Bus Selector2 : BusSelector  OutputSignals=TireFrame.omega,Steering.Wheel Angles
  Demux : Demux
  Gain : Gain  Gain=0.5
  Sum : Sum  Inputs=|++
  Terminator : Terminator
  Terminator1 : Terminator
  omega : Outport  PortDimensions=4
  SteeringWheelAngle : Outport  Port=2  PortDimensions=1
  wires:
  Bus Selector2/1 -> omega/1  "<omega>"
  Wheel/1 -> Bus Selector2/1
  Bus Selector2/2 -> Demux/1  "<Wheel Angles>"
  Demux/1 -> Sum/1
  Demux/2 -> Sum/2
  Demux/3 -> Terminator/1
  Demux/4 -> Terminator1/1
  Sum/1 -> Gain/1
  Gain/1 -> SteeringWheelAngle/1

== system ndtm_V2/Suspension/Double Wishbone Suspension ==
  Wheel : Inport
  Steering : Inport  Port=2
  Vehicle : Inport  Port=3
  Bus Creator1 : BusCreator  Inputs=5
  Bus Creator2 : BusCreator  Inputs=2
  Bus Creator3 : BusCreator  Inputs=2
  Bus Creator4 : BusCreator  Inputs=6
  Bus Selector : BusSelector  OutputSignals=z,Re,zdot,Fx,Fy,M
  Bus Selector1 : BusSelector  OutputSignals=P,V
  Independent Suspension – Double Wishbone : vehdynlibsuspension/Independent Suspension - Double Wishbone  NumAxl=2  NumTracksByAxl=[2 2]  StrgEnByAxl=[1 0]  AntiSwayEnByAxl=[1 1]  TrackNumVec="[1  2  1  2]"  AxleNumVec="[1  1  2  2]"  SuspTypesByAxle="[1  1]"  SuspImage=suspdw.png  IdealSuspEn=on  IdealSuspAxles="[1  2]"  Kz=[SUS__Compliance__cz_SpringRateFrRe_Npm__1, SUS__Compliance__cz_SpringRateFrRe_Npm__2]  F0z=[SUS__Compliance__F0z_SpringPreloadFrRe_N__1, SUS__Compliance__F0z_SpringPreloadFrRe_N__2]  Cz=[SUS__Compliance__Cz_DamperRateFrRe_Nspm__1, SUS__Compliance__Cz_DamperRateFrRe_Nspm__2]  Hmax=SUS__Compliance__Hmax_MaxHeightToHardblock_m  Toe=[SUS__Kinematics__nu0_ToeATSteerCenterFrRe_rad__1, SUS__Kinematics__nu0_ToeATSteerCenterFrRe_rad__2]  RollStrgSlp=[SUS__Kinematics__k_RollSteerVSHeightFrRe_radpm__1, SUS__Kinematics__k_RollSteerVSHeightFrRe_radpm__2]  ToeStrgSlp=SUS__Kinematics__k_ToeVSSteerF  Caster=[SUS__Kinematics__k_CasterATSteerCenterF__1, SUS__Kinematics__k_CasterATSteerCenterF__2]  CasterHslp=[SUS__Kinematics__k_CasterVSHeightFrRe__1, SUS__Kinematics__k_CasterVSHeightFrRe__2]  CasterStrgSlp=SUS__Kinematics__k_CasterVSSteerFrRe  Camber=[SUS__Kinematics__k_CamberATSteerCenterF__1, SUS__Kinematics__k_CamberATSteerCenterF__2]  CamberHslp=[SUS__Kinematics__k_CamberVSHeightFrRe__1, SUS__Kinematics__k_CamberVSHeightFrRe__2]  CamberStrgSlp=SUS__Kinematics__k_CamberVSSteerF  StrgHgtSlp=SUS__Kinematics__k_HeightVSSteerF_mprad  MappedSuspEn=off  MappedSuspAxles="[1  2]"  f_susp_axl_bp=[1 2]  f_susp_dz_bp=[-0.15 -0.14 -0.13 -0.12 -0.11 -0.10 -0.09 -0.08 -0.07 -0.06 -0.05 -0.04 -0.03 -0.02 -0.01 0.00 0.01 0.02 0.03 0.04 0.05 0.06 0.07 0.08 0.09 0.10 0.11 0.12 0.13 0.14 0.15]  f_susp_dzdot_bp=[-0.15 -0.14 -0.13 -0.12 -0.11 -0.10 -0.09 -0.08 -0.07 -0.06 -0.05 -0.04 -0.03 -0.02 -0.01 0.00 0.01 0.02 0.03 0.04 0.05 0.06 0.07 0.08 0.09 0.10 0.11 0.12 0.13 0.14 0.15]  f_susp_fmz=zeros(31,31,61,2,4)  f_susp_geom=zeros(31,61,2,3)  f_susp_strgdelta_bp=[-30,-29,-28,-27,-26,-25,-24,-23,-22,-21,-20,-19,-18,-17,-16,-15,-14,-13,-12,-11,-10,-9,-8,-7,-6,-5,-4,-3,-2,-1,0,1,2,3,4,5,6,7,8,9,10,11,12,13,14,15,16,17,18,19,20,21,22,23,24,25,26,27,28,29,30]  AntiSwayR=[SUS__Antisway__r_AntiSwayArmRadiusFrRe_m__1, SUS__Antisway__r_AntiSwayArmRadiusFrRe_m__2]  AntiSwayNtrlAng=[SUS__Antisway__phi_AntiSwayNeutralAngleFrRe_rad__1, SUS__Antisway__phi_AntiSwayNeutralAngleFrRe_rad__2]  AntiSwayTrsK=[SUS__Antisway__c_AntiSwayTSpringFrRe_Nmprad__1, SUS__Antisway__c_AntiSwayTSpringFrRe_Nmprad__2]
      settings: SourceProductName=Vehicle Dynamics Blockset  SourceProductBaseCode=VE
  Selector1 : Selector  NumberOfDimensions=2  IndexOptions=Index vector (dialog),Select all  Indices=1,1  OutputSizes=1,1
  Selector2 : Selector  NumberOfDimensions=2  IndexOptions=Index vector (dialog),Select all  Indices=2,1  OutputSizes=1,1
  Steer Rate Adapter : Subsystem
  Steering Adapter : Subsystem
  Terminator : Terminator
  Vehicle Adapter : Subsystem
  Wheel  Adapter : Subsystem
  Suspension : Outport
  wires:
  Bus Creator3/1 -> Suspension/1
  Steering Adapter/1(StrgAng) -> Independent Suspension – Double Wishbone/9
  Independent Suspension – Double Wishbone/1 -> Terminator/1  "Susp"
  Wheel  Adapter/6(Re) -> Bus Creator4/6
  Bus Selector1/1 -> Independent Suspension – Double Wishbone/7  "<P>"
  Wheel  Adapter/2(WhlFy) -> Bus Creator4/2  "Fy"
  Wheel/1 -> Wheel  Adapter/1(Wheels)
  Steer Rate Adapter/1(AngVel) -> Bus Creator1/5  "AngVel"
  Bus Creator4/1 -> Bus Selector/1
  Bus Creator2/1 -> Bus Creator3/1  "Veh"
  Independent Suspension – Double Wishbone/5 -> Selector2/1, Selector1/1  "V"
  Selector2/1 -> Bus Creator1/3  "ydot"
  Bus Selector1/2 -> Independent Suspension – Double Wishbone/8  "<V>"
  Independent Suspension – Double Wishbone/2 -> Bus Creator2/1  "F"
  Bus Selector/2 -> Independent Suspension – Double Wishbone/2  "<Re>"
  Wheel  Adapter/5(M) -> Bus Creator4/5  "M"
  Bus Selector/4 -> Independent Suspension – Double Wishbone/4  "<Fx>"
  Independent Suspension – Double Wishbone/4 -> Bus Creator1/1  "F"
  Steering/1 -> Steering Adapter/1(Steer)
  Selector1/1 -> Bus Creator1/2  "xdot"
  Independent Suspension – Double Wishbone/3 -> Bus Creator2/2  "M"
  Vehicle Adapter/1(VehSusp) -> Bus Selector1/1
  Wheel  Adapter/4(zdot) -> Bus Creator4/4
  Vehicle/1 -> Steer Rate Adapter/1(Veh), Vehicle Adapter/1(Veh)
  Bus Selector/6 -> Independent Suspension – Double Wishbone/6  "<M>"
  Bus Selector/5 -> Independent Suspension – Double Wishbone/5  "<Fy>"
  Bus Selector/1 -> Independent Suspension – Double Wishbone/1  "<z>"
  Wheel  Adapter/3(z) -> Bus Creator4/3
  Independent Suspension – Double Wishbone/6 -> Bus Creator1/4  "Ang"
  Bus Creator1/1 -> Bus Creator3/2  "Whl"
  Wheel  Adapter/1(WhlFx) -> Bus Creator4/1  "Fx"
  Bus Selector/3 -> Independent Suspension – Double Wishbone/3  "<zdot>"

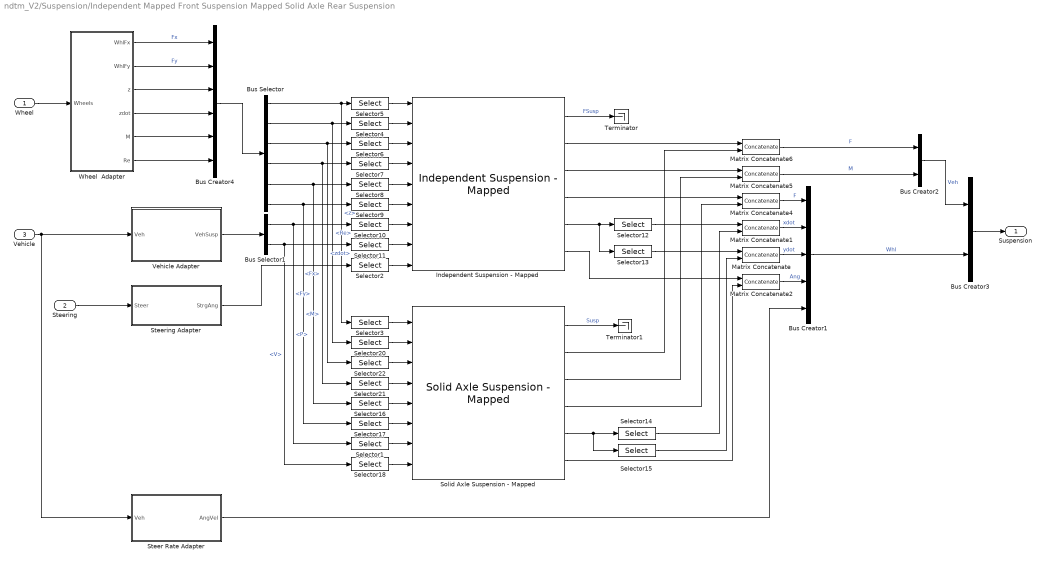
== system ndtm_V2/Suspension/Independent Mapped Front Suspension Mapped Solid Axle Rear Suspension ==
  Wheel : Inport
  Steering : Inport  Port=2
  Vehicle : Inport  Port=3
  Bus Creator1 : BusCreator  Inputs=5
  Bus Creator2 : BusCreator  Inputs=2
  Bus Creator3 : BusCreator  Inputs=2
  Bus Creator4 : BusCreator  Inputs=6
  Bus Selector : BusSelector  OutputSignals=z,Re,zdot,Fx,Fy,M
  Bus Selector1 : BusSelector  OutputSignals=P,V
  Independent Suspension - Mapped : vehdynlibsuspension/Independent Suspension - Mapped  NumAxl=1  NumTracksByAxl=2  StrgEnByAxl=1  AntiSwayEnByAxl=1  TrackNumVec="[1  2]"  AxleNumVec="[1  1]"  SuspTypesByAxle=[2]  SuspImage=suspindmap.png  IdealSuspEn=off  IdealSuspAxles="[1  2]"  Kz=64370  F0z=9810  Cz=10000  Hmax=0.5  Toe=2  RollStrgSlp=-13  ToeStrgSlp=0.01  Caster=4  CasterHslp=-13  CasterStrgSlp=0.01  Camber=4  CamberHslp=-13  CamberStrgSlp=0.01  StrgHgtSlp=0.0025  MappedSuspEn=on  MappedSuspAxles=[1]  f_susp_axl_bp=[1 2]  f_susp_dz_bp=f_susp_dz_bp  f_susp_dzdot_bp=f_susp_dzdot_bp  f_susp_fmz=f_susp_fmz  f_susp_geom=f_susp_geom  f_susp_strgdelta_bp=f_susp_strgdelta_bp  AntiSwayR=0.2  AntiSwayNtrlAng=0.5236  AntiSwayTrsK=8e2
      link override For each track and axle combination calculate suspension forces and moments/Suspension/Suspension Angle Calculations: OverrideUsingVariant=MappedSteeringEnabled
      link override For each track and axle combination calculate suspension forces and moments/Suspension/Z axis suspension characteristic: OverrideUsingVariant=MappedSuspension
      settings: SourceProductName=Vehicle Dynamics Blockset
  Matrix Concatenate{,1..2,4..6} (6 alike) : Concatenate  Mode=Multidimensional array  ConcatenateDimension=2
  Selector1 : Selector  NumberOfDimensions=2  IndexOptions=Select all,Index vector (dialog)  Indices=[1 2],[3 4]  OutputSizes=1,1
  Selector10 : Selector  NumberOfDimensions=2  IndexOptions=Select all,Index vector (dialog)  Indices=[1 2],[1 2]  OutputSizes=1,1
  Selector11 : Selector  NumberOfDimensions=2  IndexOptions=Select all,Index vector (dialog)  Indices=[1 2],[1 2]  OutputSizes=1,1
  Selector12 : Selector  NumberOfDimensions=2  InputPortWidth=3  IndexOptions=Index vector (dialog),Select all  Indices=1,1  OutputSizes=1,1
  Selector13 : Selector  NumberOfDimensions=2  InputPortWidth=3  IndexOptions=Index vector (dialog),Select all  Indices=2,1  OutputSizes=1,1
  Selector14 : Selector  NumberOfDimensions=2  InputPortWidth=3  IndexOptions=Index vector (dialog),Select all  Indices=1,1  OutputSizes=1,1
  Selector15 : Selector  NumberOfDimensions=2  InputPortWidth=3  IndexOptions=Index vector (dialog),Select all  Indices=2,1  OutputSizes=1,1
  Selector{3,16,20..22} (5 alike) : Selector  IndexOptions=Index vector (dialog)  Indices=[3 4]  OutputSizes=1
  Selector17 : Selector  NumberOfDimensions=2  IndexOptions=Select all,Index vector (dialog)  Indices=[1 2],[3 4]  OutputSizes=1,1
  Selector18 : Selector  NumberOfDimensions=2  IndexOptions=Select all,Index vector (dialog)  Indices=[1 2],[3 4]  OutputSizes=1,1
  Selector{2,4..8} (6 alike) : Selector  IndexOptions=Index vector (dialog)  Indices=[1 2]  OutputSizes=1
  Selector9 : Selector  NumberOfDimensions=2  IndexOptions=Select all,Index vector (dialog)  Indices=[1 2],[1 2]  OutputSizes=1,1
  Solid Axle Suspension - Mapped : vehdynlibsuspension/Solid Axle Suspension - Mapped  NumAxl=1  NumTracksByAxl=2  StrgEnByAxl=0  TrackNumVec="[1  2]"  AxleNumVec="[1  1]"  SuspTypesByAxle=[2]  SuspImage=suspsamap.png  AxlIxx=AxlIxx  AxlM=AxlM  TrackCoords=[0 0;VEH.TrackWidth*[-1 1]/2;0 0]  SuspCoords=[0 0;VEH.TrackWidth*[-1 1]/2;0 0]  KzWhlAxl=KzWhlAxl  F0zWhlAxl=F0zWhlAxl  CzWhlAxl=CzWhlAxl  IdealSuspEn=off  IdealSuspAxles="[1  2]"  Kz=64370  F0z=9810  Cz=10000  Hmax=0.5  Toe=2  RollStrgSlp=-13  ToeStrgSlp=0.01  Caster=4  CasterHslp=-13  CasterStrgSlp=0.01  Camber=4  CamberHslp=-13  CamberStrgSlp=0.01  StrgHgtSlp=0.0025  MappedSuspEn=on  MappedSuspAxles=[1]  f_susp_axl_bp=[1 2]  f_susp_dz_bp=f_susp_dz_bp  f_susp_dzdot_bp=f_susp_dzdot_bp  f_susp_fmz=f_susp_fmz  f_susp_geom=f_susp_geom  f_susp_strgdelta_bp=f_susp_strgdelta_bp
      link override For each track and axle combination calculate suspension forces and moments/Suspension/Suspension Angle Calculations: OverrideUsingVariant=MappedSteeringEnabled
      link override For each track and axle combination calculate suspension forces and moments/Suspension/Z axis suspension characteristic: OverrideUsingVariant=MappedSuspension
      settings: SourceProductName=Vehicle Dynamics Blockset
  Steer Rate Adapter : Subsystem
  Steering Adapter : Subsystem
  Terminator : Terminator
  Terminator1 : Terminator
  Vehicle Adapter : Subsystem
  Wheel  Adapter : Subsystem
  Suspension : Outport
  wires:
  Solid Axle Suspension - Mapped/5 -> Selector15/1, Selector14/1
  Selector22/1 -> Solid Axle Suspension - Mapped/3
  Bus Selector/3 -> Selector22/1, Selector6/1  "<zdot>"
  Solid Axle Suspension - Mapped/4 -> Matrix Concatenate4/2
  Solid Axle Suspension - Mapped/1 -> Terminator1/1  "Susp"
  Selector12/1 -> Matrix Concatenate1/1
  Selector7/1 -> Independent Suspension - Mapped/4
  Selector18/1 -> Solid Axle Suspension - Mapped/8
  Selector13/1 -> Matrix Concatenate/1
  Selector14/1 -> Matrix Concatenate1/2
  Selector21/1 -> Solid Axle Suspension - Mapped/4
  Vehicle/1 -> Steer Rate Adapter/1(Veh), Vehicle Adapter/1(Veh)
  Wheel  Adapter/4(zdot) -> Bus Creator4/4
  Solid Axle Suspension - Mapped/3 -> Matrix Concatenate5/2
  Selector1/1 -> Solid Axle Suspension - Mapped/7
  Matrix Concatenate4/1 -> Bus Creator1/1  "F"
  Selector16/1 -> Solid Axle Suspension - Mapped/5
  Matrix Concatenate5/1 -> Bus Creator2/2  "M"
  Independent Suspension - Mapped/4 -> Matrix Concatenate4/1
  Selector4/1 -> Independent Suspension - Mapped/2
  Selector10/1 -> Independent Suspension - Mapped/7
  Selector9/1 -> Independent Suspension - Mapped/6
  Wheel  Adapter/3(z) -> Bus Creator4/3
  Solid Axle Suspension - Mapped/2 -> Matrix Concatenate6/2
  Wheel/1 -> Wheel  Adapter/1(Wheels)
  Selector5/1 -> Independent Suspension - Mapped/1
  Independent Suspension - Mapped/3 -> Matrix Concatenate5/1
  Selector8/1 -> Independent Suspension - Mapped/5
  Independent Suspension - Mapped/2 -> Matrix Concatenate6/1
  Independent Suspension - Mapped/6 -> Matrix Concatenate2/1
  Selector20/1 -> Solid Axle Suspension - Mapped/2
  Independent Suspension - Mapped/1 -> Terminator/1  "FSusp"
  Bus Creator2/1 -> Bus Creator3/1  "Veh"
  Bus Selector/4 -> Selector7/1, Selector21/1  "<Fx>"
  Independent Suspension - Mapped/5 -> Selector12/1, Selector13/1
  Matrix Concatenate2/1 -> Bus Creator1/4  "Ang"
  Wheel  Adapter/2(WhlFy) -> Bus Creator4/2  "Fy"
  Bus Creator4/1 -> Bus Selector/1
  Selector17/1 -> Solid Axle Suspension - Mapped/6
  Selector2/1 -> Independent Suspension - Mapped/9
  Wheel  Adapter/5(M) -> Bus Creator4/5
  Matrix Concatenate/1 -> Bus Creator1/3  "ydot"
  Steering/1 -> Steering Adapter/1(Steer)
  Matrix Concatenate1/1 -> Bus Creator1/2  "xdot"
  Selector15/1 -> Matrix Concatenate/2
  Selector3/1 -> Solid Axle Suspension - Mapped/1
  Bus Selector1/2 -> Selector11/1, Selector18/1  "<V>"
  Vehicle Adapter/1(VehSusp) -> Bus Selector1/1
  Steering Adapter/1(StrgAng) -> Selector2/1
  Selector6/1 -> Independent Suspension - Mapped/3
  Bus Selector/6 -> Selector9/1, Selector17/1  "<M>"
  Wheel  Adapter/1(WhlFx) -> Bus Creator4/1  "Fx"
  Selector11/1 -> Independent Suspension - Mapped/8
  Wheel  Adapter/6(Re) -> Bus Creator4/6
  Matrix Concatenate6/1 -> Bus Creator2/1  "F"
  Bus Selector1/1 -> Selector10/1, Selector1/1  "<P>"
  Solid Axle Suspension - Mapped/6 -> Matrix Concatenate2/2
  Bus Selector/1 -> Selector3/1, Selector5/1  "<z>"
  Bus Selector/5 -> Selector8/1, Selector16/1  "<Fy>"
  Bus Creator1/1 -> Bus Creator3/2  "Whl"
  Bus Creator3/1 -> Suspension/1
  Bus Selector/2 -> Selector20/1, Selector4/1  "<Re>"
  Steer Rate Adapter/1(AngVel) -> Bus Creator1/5

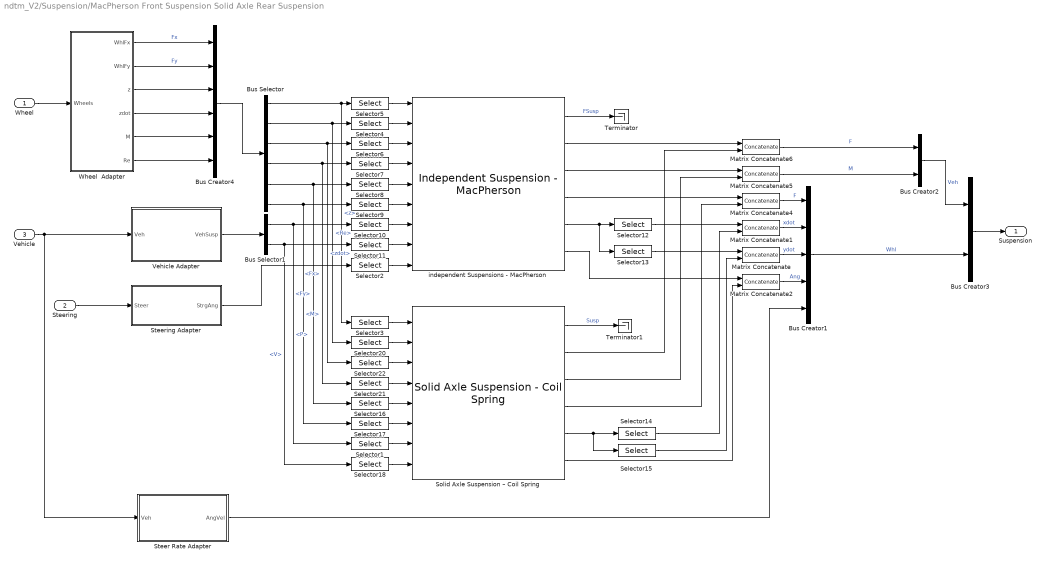
== system ndtm_V2/Suspension/MacPherson Front Suspension Solid Axle Rear Suspension ==
  Wheel : Inport
  Steering : Inport  Port=2
  Vehicle : Inport  Port=3
  Bus Creator1 : BusCreator  Inputs=5
  Bus Creator2 : BusCreator  Inputs=2
  Bus Creator3 : BusCreator  Inputs=2
  Bus Creator4 : BusCreator  Inputs=6
  Bus Selector : BusSelector  OutputSignals=z,Re,zdot,Fx,Fy,M
  Bus Selector1 : BusSelector  OutputSignals=P,V
  Matrix Concatenate{,1..2,4..6} (6 alike) : Concatenate  Mode=Multidimensional array  ConcatenateDimension=2
  Selector1 : Selector  NumberOfDimensions=2  IndexOptions=Select all,Index vector (dialog)  Indices=[1 2],[3 4]  OutputSizes=1,1
  Selector10 : Selector  NumberOfDimensions=2  IndexOptions=Select all,Index vector (dialog)  Indices=[1 2],[1 2]  OutputSizes=1,1
  Selector11 : Selector  NumberOfDimensions=2  IndexOptions=Select all,Index vector (dialog)  Indices=[1 2],[1 2]  OutputSizes=1,1
  Selector12 : Selector  NumberOfDimensions=2  InputPortWidth=3  IndexOptions=Index vector (dialog),Select all  Indices=1,1  OutputSizes=1,1
  Selector13 : Selector  NumberOfDimensions=2  InputPortWidth=3  IndexOptions=Index vector (dialog),Select all  Indices=2,1  OutputSizes=1,1
  Selector14 : Selector  NumberOfDimensions=2  InputPortWidth=3  IndexOptions=Index vector (dialog),Select all  Indices=1,1  OutputSizes=1,1
  Selector15 : Selector  NumberOfDimensions=2  InputPortWidth=3  IndexOptions=Index vector (dialog),Select all  Indices=2,1  OutputSizes=1,1
  Selector{3,16,20..22} (5 alike) : Selector  IndexOptions=Index vector (dialog)  Indices=[3 4]  OutputSizes=1
  Selector17 : Selector  NumberOfDimensions=2  IndexOptions=Select all,Index vector (dialog)  Indices=[1 2],[3 4]  OutputSizes=1,1
  Selector18 : Selector  NumberOfDimensions=2  IndexOptions=Select all,Index vector (dialog)  Indices=[1 2],[3 4]  OutputSizes=1,1
  Selector{2,4..8} (6 alike) : Selector  IndexOptions=Index vector (dialog)  Indices=[1 2]  OutputSizes=1
  Selector9 : Selector  NumberOfDimensions=2  IndexOptions=Select all,Index vector (dialog)  Indices=[1 2],[1 2]  OutputSizes=1,1
  Solid Axle Suspension – Coil Spring : vehdynlibsuspension/Solid Axle Suspension - Coil Spring  NumAxl=1  NumTracksByAxl=2  StrgEnByAxl=0  TrackNumVec="[1  2]"  AxleNumVec="[1  1]"  SuspTypesByAxle=[1]  SuspImage=suspsacoil.png  AxlIxx=AxlIxx  AxlM=AxlM  TrackCoords=[0 0;VEH.TrackWidth*[-1 1]/2;0 0]  SuspCoords=[0 0;VEH.TrackWidth*[-1 1]/2;0 0]  KzWhlAxl=KzWhlAxl  F0zWhlAxl=F0zWhlAxl  CzWhlAxl=CzWhlAxl  IdealSuspEn=on  IdealSuspAxles=[1]  Kz=Kz  F0z=F0z(2)  Cz=Cz  Hmax=Hmax  Toe=0.  RollStrgSlp=0.  ToeStrgSlp=0  Caster=0.  CasterHslp=0.  CasterStrgSlp=0.01  Camber=0.  CamberHslp=0.  CamberStrgSlp=0.01  StrgHgtSlp=0.1432  MappedSuspEn=off  MappedSuspAxles="[1  2]"  f_susp_axl_bp=[1 2]  f_susp_dz_bp=[-0.15 -0.14 -0.13 -0.12 -0.11 -0.10 -0.09 -0.08 -0.07 -0.06 -0.05 -0.04 -0.03 -0.02 -0.01 0.00 0.01 0.02 0.03 0.04 0.05 0.06 0.07 0.08 0.09 0.10 0.11 0.12 0.13 0.14 0.15]  f_susp_dzdot_bp=[-0.15 -0.14 -0.13 -0.12 -0.11 -0.10 -0.09 -0.08 -0.07 -0.06 -0.05 -0.04 -0.03 -0.02 -0.01 0.00 0.01 0.02 0.03 0.04 0.05 0.06 0.07 0.08 0.09 0.10 0.11 0.12 0.13 0.14 0.15]  f_susp_fmz=zeros(31,31,61,2,4)  f_susp_geom=zeros(31,61,2,3)  f_susp_strgdelta_bp=[-30,-29,-28,-27,-26,-25,-24,-23,-22,-21,-20,-19,-18,-17,-16,-15,-14,-13,-12,-11,-10,-9,-8,-7,-6,-5,-4,-3,-2,-1,0,1,2,3,4,5,6,7,8,9,10,11,12,13,14,15,16,17,18,19,20,21,22,23,24,25,26,27,28,29,30]
      settings: SourceProductName=Vehicle Dynamics Blockset  SourceProductBaseCode=VE
  Steer Rate Adapter : Subsystem
  Steering Adapter : Subsystem
  Terminator : Terminator
  Terminator1 : Terminator
  Vehicle Adapter : Subsystem
  Wheel  Adapter : Subsystem
  independent Suspensions - MacPherson : vehdynlibsuspension/Independent Suspension - MacPherson  NumAxl=1  NumTracksByAxl=2  StrgEnByAxl=1  AntiSwayEnByAxl=1  TrackNumVec="[1  2]"  AxleNumVec="[1  1]"  SuspTypesByAxle=[1]  SuspImage=suspmacp.png  IdealSuspEn=on  IdealSuspAxles=[1]  Kz=Kz  F0z=F0z(1)  Cz=Cz  Hmax=Hmax  Toe=0.  RollStrgSlp=0.  ToeStrgSlp=0.  Caster=0.  CasterHslp=0.  CasterStrgSlp=0.  Camber=0.  CamberHslp=0.  CamberStrgSlp=0.  StrgHgtSlp=0.1432  MappedSuspEn=off  MappedSuspAxles="[1  2]"  f_susp_axl_bp=[1 2]  f_susp_dz_bp=[-0.15 -0.14 -0.13 -0.12 -0.11 -0.10 -0.09 -0.08 -0.07 -0.06 -0.05 -0.04 -0.03 -0.02 -0.01 0.00 0.01 0.02 0.03 0.04 0.05 0.06 0.07 0.08 0.09 0.10 0.11 0.12 0.13 0.14 0.15]  f_susp_dzdot_bp=[-0.15 -0.14 -0.13 -0.12 -0.11 -0.10 -0.09 -0.08 -0.07 -0.06 -0.05 -0.04 -0.03 -0.02 -0.01 0.00 0.01 0.02 0.03 0.04 0.05 0.06 0.07 0.08 0.09 0.10 0.11 0.12 0.13 0.14 0.15]  f_susp_fmz=zeros(31,31,61,2,4)  f_susp_geom=zeros(31,61,2,3)  f_susp_strgdelta_bp=[-30,-29,-28,-27,-26,-25,-24,-23,-22,-21,-20,-19,-18,-17,-16,-15,-14,-13,-12,-11,-10,-9,-8,-7,-6,-5,-4,-3,-2,-1,0,1,2,3,4,5,6,7,8,9,10,11,12,13,14,15,16,17,18,19,20,21,22,23,24,25,26,27,28,29,30]  AntiSwayR=0.2  AntiSwayNtrlAng=0.5236  AntiSwayTrsK=8e+02
      settings: SourceProductName=Vehicle Dynamics Blockset  SourceProductBaseCode=VE
  Suspension : Outport
  wires:
  Bus Creator3/1 -> Suspension/1
  Bus Creator1/1 -> Bus Creator3/2  "Whl"
  Bus Selector1/2 -> Selector11/1, Selector18/1  "<V>"
  Bus Selector/6 -> Selector9/1, Selector17/1  "<M>"
  Bus Selector/5 -> Selector8/1, Selector16/1  "<Fy>"
  Bus Selector/1 -> Selector3/1, Selector5/1  "<z>"
  Steering/1 -> Steering Adapter/1(Steer)
  Bus Selector1/1 -> Selector10/1, Selector1/1  "<P>"
  Matrix Concatenate/1 -> Bus Creator1/3  "ydot"
  independent Suspensions - MacPherson/5 -> Selector12/1, Selector13/1
  independent Suspensions - MacPherson/6 -> Matrix Concatenate2/1
  Selector12/1 -> Matrix Concatenate1/1
  independent Suspensions - MacPherson/4 -> Matrix Concatenate4/1
  independent Suspensions - MacPherson/1 -> Terminator/1  "FSusp"
  Bus Selector/4 -> Selector7/1, Selector21/1  "<Fx>"
  Vehicle Adapter/1(VehSusp) -> Bus Selector1/1
  independent Suspensions - MacPherson/2 -> Matrix Concatenate6/1
  independent Suspensions - MacPherson/3 -> Matrix Concatenate5/1
  Bus Creator2/1 -> Bus Creator3/1  "Veh"
  Steering Adapter/1(StrgAng) -> Selector2/1
  Bus Creator4/1 -> Bus Selector/1
  Wheel  Adapter/2(WhlFy) -> Bus Creator4/2  "Fy"
  Wheel  Adapter/1(WhlFx) -> Bus Creator4/1  "Fx"
  Wheel/1 -> Wheel  Adapter/1(Wheels)
  Wheel  Adapter/3(z) -> Bus Creator4/3
  Wheel  Adapter/4(zdot) -> Bus Creator4/4
  Wheel  Adapter/5(M) -> Bus Creator4/5
  Bus Selector/2 -> Selector20/1, Selector4/1  "<Re>"
  Selector2/1 -> independent Suspensions - MacPherson/9
  Selector3/1 -> Solid Axle Suspension – Coil Spring/1
  Selector4/1 -> independent Suspensions - MacPherson/2
  Selector5/1 -> independent Suspensions - MacPherson/1
  Selector6/1 -> independent Suspensions - MacPherson/3
  Selector7/1 -> independent Suspensions - MacPherson/4
  Selector8/1 -> independent Suspensions - MacPherson/5
  Selector9/1 -> independent Suspensions - MacPherson/6
  Selector10/1 -> independent Suspensions - MacPherson/7
  Selector11/1 -> independent Suspensions - MacPherson/8
  Selector13/1 -> Matrix Concatenate/1
  Selector15/1 -> Matrix Concatenate/2
  Matrix Concatenate1/1 -> Bus Creator1/2  "xdot"
  Selector14/1 -> Matrix Concatenate1/2
  Matrix Concatenate2/1 -> Bus Creator1/4  "Ang"
  Solid Axle Suspension – Coil Spring/6 -> Matrix Concatenate2/2
  Matrix Concatenate4/1 -> Bus Creator1/1  "F"
  Solid Axle Suspension – Coil Spring/4 -> Matrix Concatenate4/2
  Matrix Concatenate5/1 -> Bus Creator2/2  "M"
  Matrix Concatenate6/1 -> Bus Creator2/1  "F"
  Solid Axle Suspension – Coil Spring/2 -> Matrix Concatenate6/2
  Selector16/1 -> Solid Axle Suspension – Coil Spring/5
  Selector17/1 -> Solid Axle Suspension – Coil Spring/6
  Selector1/1 -> Solid Axle Suspension – Coil Spring/7
  Selector18/1 -> Solid Axle Suspension – Coil Spring/8
  Selector20/1 -> Solid Axle Suspension – Coil Spring/2
  Wheel  Adapter/6(Re) -> Bus Creator4/6
  Selector21/1 -> Solid Axle Suspension – Coil Spring/4
  Solid Axle Suspension – Coil Spring/3 -> Matrix Concatenate5/2
  Vehicle/1 -> Steer Rate Adapter/1(Veh), Vehicle Adapter/1(Veh)
  Selector22/1 -> Solid Axle Suspension – Coil Spring/3
  Bus Selector/3 -> Selector22/1, Selector6/1  "<zdot>"
  Solid Axle Suspension – Coil Spring/1 -> Terminator1/1  "Susp"
  Solid Axle Suspension – Coil Spring/5 -> Selector15/1, Selector14/1
  Steer Rate Adapter/1(AngVel) -> Bus Creator1/5
